simulink model "VSCHVDCunit"  (R2025b)
settings: Solver=VariableStepAuto  StartTime=0.0  StopTime=5  RelTol=1e-3
PreLoadFcn:
  | HVDCParameters;
undefined symbols (not defined in the file): Connection1, Connection2, Connection3, DiscIntNeverNeededParam, ee_sli_rtmsupport, frt, gcbh, grid, HVDC, lvrt, pll, pmsm, PVController, time, Ts, Vdcs0, windController, windTransformer, windTurbine
libraries: nesl_utility x25, fl_lib x24, ee_lib x13, eeGeneralControl x4, eeTransforms x3, simulink x3
(part 1 of 2)
settings Model: SimulationMode=accelerator  Creator=Rajarshi  LastModifiedBy=rajarshd

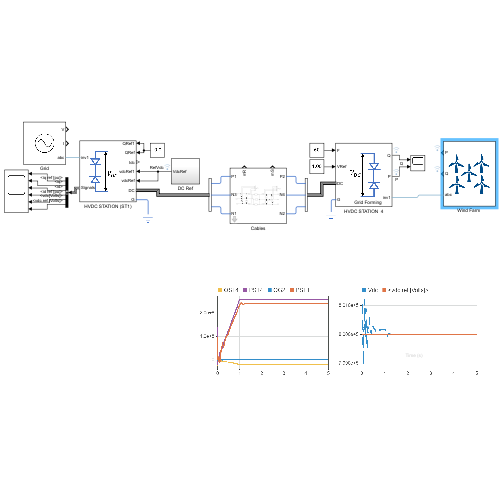
[thumbnail: Simulink's stored preview of the top-level diagram]
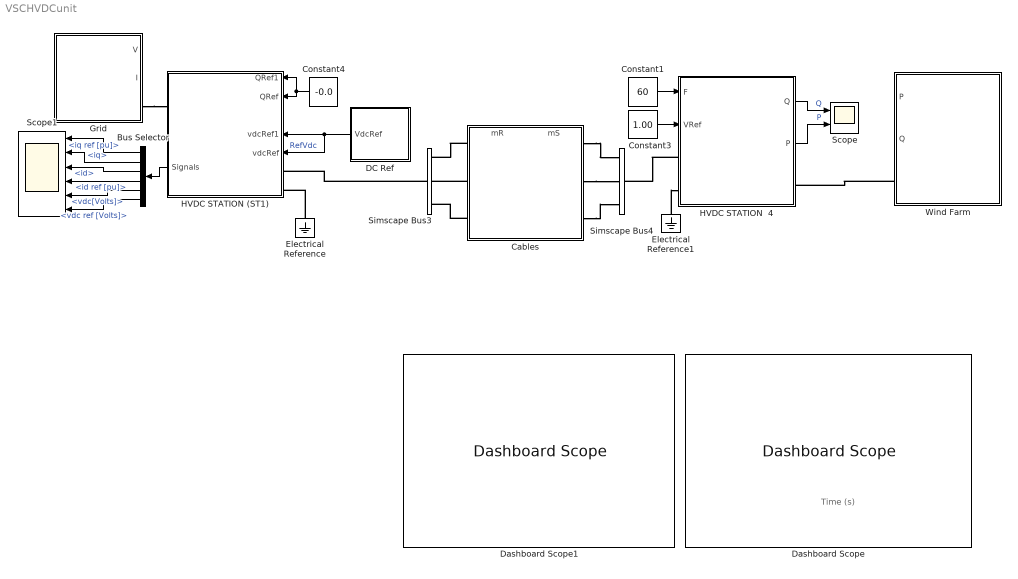
== system VSCHVDCunit ==
  note: Time (s)
  Bus Selector : BusSelector  OutputSignals=iq ref [pu],iq,id,id ref [pu],vdc[Volts],vdc ref [Volts]
  Cables : Subsystem
      settings: PortSchema="{\"entries\":[{\"content\":{\"sides\":[{\"content\":{\"connectorIds\":[\"LConn1\",\"LConn2\",\"LConn3\"]},\"type\":\"ConnectorPlacement.EquallySpacedRectSide\",\"uuid\":\"66d4cfbf-dcba-4749-bf5d-5811a775276e\"},{\"content\":{\"connectorIds\":[\"RConn1\",\"RConn2\",\"RConn3\"],\"side\":\"RIGHT\"},\"type\":\"ConnectorPlacement.EquallySpacedRectSide\",\"uuid\":\"35abdffa-cda0-46f2-9903-3f86a9532248\"},{\"content\":{\"connectorIds\":[\"Out1\",\"Out2\"],\"side\":\"TOP\"},\"type\":\"ConnectorPlacement.EquallySpacedRectSide\",\"uuid\":\"3c5502e5-1b76-444d-b26b-a5789383a319\"},{\"content\":{\"side\":\"BOTTOM\"},\"type\":\"ConnectorPlacement.EquallySpacedRectSide\",\"uuid\":\"683abed6-51b1-463c-bfde-96cc94cb06b2\"}]},\"type\":\"ConnectorPlacement.EquallySpacedConnector\",\"uuid\":\"b78b2c4f-7eb3-43f3-aa61-891430661a3a\"}],\"packageUris\":[\"http://schema.mathworks.com/mf0/Connector/R2020b\"],\"version\":\"1.0\"}"
  Constant1 : Constant  Value=60
  Constant3 : Constant  Value=1.00
  Constant4 : Constant  Value=-0.0
  DC Ref : Subsystem
  Dashboard Scope : DashboardScope  FontColor=[0.0, 0.0, 0.0]
  Dashboard Scope1 : DashboardScope  FontColor=[0.0, 0.0, 0.0]
  Electrical Reference : fl_lib/Electrical/Electrical Elements/Electrical Reference
  Electrical Reference1 : fl_lib/Electrical/Electrical Elements/Electrical Reference
  Grid : Subsystem
  HVDC STATION  4 : Subsystem
      mask Display:
      | text(40,10, 'Grid Forming');
      | image('HVDCstation.png', [0,0,0,0,80,80]);
  HVDC STATION (ST1) : Subsystem
      settings: PortSchema="{\"entries\":[{\"content\":{\"sides\":[{\"content\":{\"connectorIds\":[\"In1\",\"In2\",\"LConn1\",\"In3\",\"In4\",\"LConn2\",\"LConn3\"]},\"type\":\"ConnectorPlacement.EquallySpacedRectSide\",\"uuid\":\"825870e3-6597-48fb-b44e-9cac78187e1c\"},{\"content\":{\"connectorIds\":[\"RConn1\",\"Out1\"],\"side\":\"RIGHT\"},\"type\":\"ConnectorPlacement.EquallySpacedRectSide\",\"uuid\":\"0ccf2e17-8e04-4158-8531-c061fa3c835c\"},{\"content\":{\"side\":\"TOP\"},\"type\":\"ConnectorPlacement.EquallySpacedRectSide\",\"uuid\":\"f5f3d6c6-bb99-4c25-841e-4b6e2b2ba3c2\"}]},\"type\":\"ConnectorPlacement.EquallySpacedConnector\",\"uuid\":\"7882ba9b-b66e-421c-89fd-6c0e858bc84c\"}],\"packageUris\":[\"http://schema.mathworks.com/mf0/Connector/R2020b\"],\"version\":\"1.0\"}"
      mask Display: image('HVDCstation1.png', [0,2,12,2,80,80]);
  Scope : Scope  NumInputPorts=2
      settings: ActiveDisplayYMinimum=-8.229856003977344E+8  ActiveDisplayYMaximum=7.0866847199803662E+8
  Scope1 : Scope  NumInputPorts=6
      settings: ActiveDisplayYMinimum=-0.01126  ActiveDisplayYMaximum=0.00125
  Simscape Bus3 : SimscapeBus  HierarchyStrings=Connection1;Connection2;Connection3
  Simscape Bus4 : SimscapeBus  HierarchyStrings=Connection1;Connection2;Connection3
  "Wind Farm " : Subsystem
      mask Display: image('Windfirm3.png', [0,0,0,0,80,80]);
  wires:
  DC Ref/1(VdcRef) -> HVDC STATION (ST1)/4(vdcRef), HVDC STATION (ST1)/3(vdcRef1)  "RefVdc"
  Constant1/1 -> HVDC STATION  4/1(F)
  Constant4/1 -> HVDC STATION (ST1)/1(QRef1), HVDC STATION (ST1)/2(QRef)
  Constant3/1 -> HVDC STATION  4/2(VRef)
  HVDC STATION (ST1)/1(Signals) -> Bus Selector/1
  Bus Selector/1 -> Scope1/1  "<iq ref [pu]>"
  Bus Selector/2 -> Scope1/2  "<iq>"
  Bus Selector/3 -> Scope1/3  "<id>"
  Bus Selector/4 -> Scope1/4  "<id ref [pu]>"
  Bus Selector/5 -> Scope1/5  "<vdc[Volts]>"
  Bus Selector/6 -> Scope1/6  "<vdc ref [Volts]>"
  HVDC STATION  4/1(Q) -> Scope/1  "Q"
  HVDC STATION  4/2(P) -> Scope/2  "P"
  connections:
  Grid/RConn1 -- HVDC STATION (ST1)/RConn1
  "Wind Farm "/RConn1 -- HVDC STATION  4/RConn1
  Cables/RConn3 -- Simscape Bus4/LConn3
  Cables/LConn1 -- Simscape Bus3/LConn1
  Cables/LConn3 -- Simscape Bus3/LConn3
  Cables/LConn2 -- Simscape Bus3/LConn2
  Cables/RConn2 -- Simscape Bus4/LConn2
  Cables/RConn1 -- Simscape Bus4/LConn1
  HVDC STATION  4/LConn1 -- Simscape Bus4/RConn1
  Simscape Bus3/RConn1 -- HVDC STATION (ST1)/LConn2
  Electrical Reference/LConn1 -- HVDC STATION (ST1)/LConn3
  Electrical Reference1/LConn1 -- HVDC STATION  4/LConn2

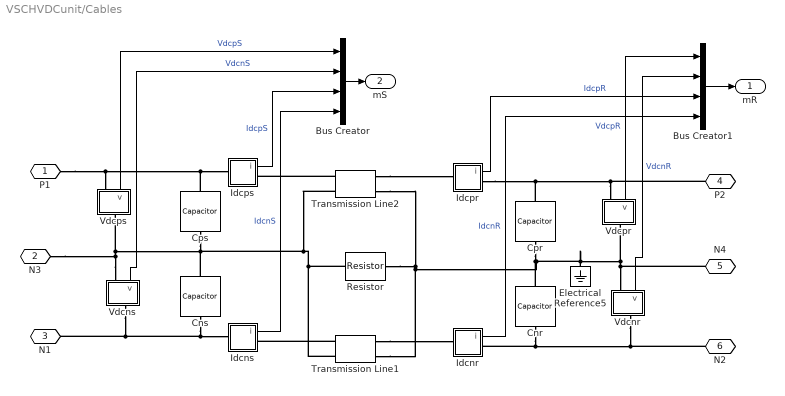
== system VSCHVDCunit/Cables ==
  Bus Creator : BusCreator  Inputs=4
  Bus Creator1 : BusCreator  Inputs=4
  Cnr : fl_lib/Electrical/Electrical Elements/Capacitor  c=0.1e-6 F  r=0 Ohm  g=0 1/Ohm  i_specify=off  i_priority=High  i=0 A  i_nominal_specify=off  i_nominal_value=1  i_nominal_unit=A  v_specify=off  v_priority=High  v=Vdcs0/2 V  v_nominal_specify=off  v_nominal_value=1  v_nominal_unit=V  vc_specify=on  vc_priority=High  vc=HVDC.Vdc V  vc_nominal_specify=off  vc_nominal_value=1  vc_nominal_unit=V
  Cns : fl_lib/Electrical/Electrical Elements/Capacitor  c=0.1e-6 F  r=0 Ohm  g=0 1/Ohm  i_specify=off  i_priority=High  i=0 A  i_nominal_specify=off  i_nominal_value=1  i_nominal_unit=A  v_specify=off  v_priority=High  v=Vdcs0/2 V  v_nominal_specify=off  v_nominal_value=1  v_nominal_unit=V  vc_specify=on  vc_priority=High  vc=HVDC.Vdc V  vc_nominal_specify=off  vc_nominal_value=1  vc_nominal_unit=V
  Cpr : fl_lib/Electrical/Electrical Elements/Capacitor  c=0.1e-6 F  r=0 Ohm  g=0 1/Ohm  i_specify=off  i_priority=High  i=0 A  i_nominal_specify=off  i_nominal_value=1  i_nominal_unit=A  v_specify=off  v_priority=High  v=Vdcs0/2 V  v_nominal_specify=off  v_nominal_value=1  v_nominal_unit=V  vc_specify=on  vc_priority=High  vc=HVDC.Vdc V  vc_nominal_specify=off  vc_nominal_value=1  vc_nominal_unit=V
  Cps : fl_lib/Electrical/Electrical Elements/Capacitor  c=0.1e-6 F  r=0 Ohm  g=0 1/Ohm  i_specify=off  i_priority=High  i=0 A  i_nominal_specify=off  i_nominal_value=1  i_nominal_unit=A  v_specify=off  v_priority=High  v=Vdcs0/2 V  v_nominal_specify=off  v_nominal_value=1  v_nominal_unit=V  vc_specify=on  vc_priority=High  vc=HVDC.Vdc V  vc_nominal_specify=off  vc_nominal_value=1  vc_nominal_unit=V
  Electrical Reference5 : fl_lib/Electrical/Electrical Elements/Electrical Reference
  Idcnr : Subsystem
      settings: PortSchema="{\"entries\":[{\"content\":{\"sides\":[{\"content\":{\"connectorIds\":[\"LConn1\"]},\"type\":\"ConnectorPlacement.EquallySpacedRectSide\",\"uuid\":\"b182dbc5-c8d5-4832-a7cd-ea3787954646\"},{\"content\":{\"connectorIds\":[\"RConn1\",\"Out1\"],\"side\":\"RIGHT\"},\"type\":\"ConnectorPlacement.EquallySpacedRectSide\",\"uuid\":\"bfc6f163-1abf-440b-aa89-1443f971fd07\"},{\"content\":{\"connectorIds\":[],\"side\":\"TOP\"},\"type\":\"ConnectorPlacement.EquallySpacedRectSide\",\"uuid\":\"dd2a104c-9a72-483e-91c4-dbef9b359450\"}]},\"type\":\"ConnectorPlacement.EquallySpacedConnector\",\"uuid\":\"ce98cc3b-f524-409d-a465-fff2e3b7df79\"}],\"packageUris\":[\"http://schema.mathworks.com/mf0/Connector/R2020b\"],\"version\":\"1.0\"}"
  Idcns : Subsystem
      settings: PortSchema="{\"entries\":[{\"content\":{\"sides\":[{\"content\":{\"connectorIds\":[\"LConn1\"]},\"type\":\"ConnectorPlacement.EquallySpacedRectSide\",\"uuid\":\"b182dbc5-c8d5-4832-a7cd-ea3787954646\"},{\"content\":{\"connectorIds\":[\"RConn1\",\"Out1\"],\"side\":\"RIGHT\"},\"type\":\"ConnectorPlacement.EquallySpacedRectSide\",\"uuid\":\"bfc6f163-1abf-440b-aa89-1443f971fd07\"},{\"content\":{\"connectorIds\":[],\"side\":\"TOP\"},\"type\":\"ConnectorPlacement.EquallySpacedRectSide\",\"uuid\":\"dd2a104c-9a72-483e-91c4-dbef9b359450\"}]},\"type\":\"ConnectorPlacement.EquallySpacedConnector\",\"uuid\":\"ce98cc3b-f524-409d-a465-fff2e3b7df79\"}],\"packageUris\":[\"http://schema.mathworks.com/mf0/Connector/R2020b\"],\"version\":\"1.0\"}"
  Idcpr : Subsystem
      settings: PortSchema="{\"entries\":[{\"content\":{\"sides\":[{\"content\":{\"connectorIds\":[\"LConn1\"]},\"type\":\"ConnectorPlacement.EquallySpacedRectSide\",\"uuid\":\"b182dbc5-c8d5-4832-a7cd-ea3787954646\"},{\"content\":{\"connectorIds\":[\"RConn1\",\"Out1\"],\"side\":\"RIGHT\"},\"type\":\"ConnectorPlacement.EquallySpacedRectSide\",\"uuid\":\"bfc6f163-1abf-440b-aa89-1443f971fd07\"},{\"content\":{\"connectorIds\":[],\"side\":\"TOP\"},\"type\":\"ConnectorPlacement.EquallySpacedRectSide\",\"uuid\":\"dd2a104c-9a72-483e-91c4-dbef9b359450\"}]},\"type\":\"ConnectorPlacement.EquallySpacedConnector\",\"uuid\":\"ce98cc3b-f524-409d-a465-fff2e3b7df79\"}],\"packageUris\":[\"http://schema.mathworks.com/mf0/Connector/R2020b\"],\"version\":\"1.0\"}"
  Idcps : Subsystem
      settings: PortSchema="{\"entries\":[{\"content\":{\"sides\":[{\"content\":{\"connectorIds\":[\"LConn1\"]},\"type\":\"ConnectorPlacement.EquallySpacedRectSide\",\"uuid\":\"b182dbc5-c8d5-4832-a7cd-ea3787954646\"},{\"content\":{\"connectorIds\":[\"RConn1\",\"Out1\"],\"side\":\"RIGHT\"},\"type\":\"ConnectorPlacement.EquallySpacedRectSide\",\"uuid\":\"bfc6f163-1abf-440b-aa89-1443f971fd07\"},{\"content\":{\"connectorIds\":[],\"side\":\"TOP\"},\"type\":\"ConnectorPlacement.EquallySpacedRectSide\",\"uuid\":\"dd2a104c-9a72-483e-91c4-dbef9b359450\"}]},\"type\":\"ConnectorPlacement.EquallySpacedConnector\",\"uuid\":\"ce98cc3b-f524-409d-a465-fff2e3b7df79\"}],\"packageUris\":[\"http://schema.mathworks.com/mf0/Connector/R2020b\"],\"version\":\"1.0\"}"
  Resistor : fl_lib/Electrical/Electrical Elements/Resistor  R=125*1e-5 Ohm  i_specify=off  i_priority=None  i=0 A  i_nominal_specify=off  i_nominal_value=1  i_nominal_unit=A  v_specify=off  v_priority=None  v=0 V  v_nominal_specify=off  v_nominal_value=1  v_nominal_unit=V
  Transmission Line1 : ee_lib/Passive/Lines/Transmission Line  model_type=4  TD=5 ns  LC_param=2  Z0_delay_based=50 Ohm  Z0=50 Ohm  freq=60 Hz  Ll=0.47/1000 mH/m  L=2.1120/1000 mH/m  C=0.1906/1000 uF/m  R=0.0095/1000 Ohm/m  G=0.048 /1000 uS/m  LEN=125 km  N=1
      settings: InternalSimscapePortConfiguration="{\"Bottom\":[],\"Left\":[{\"id\":\"p1\",\"label\":\"\",\"type\":\"foundation.electrical.electrical\"},{\"id\":\"n1\",\"label\":\"\",\"type\":\"foundation.electrical.electrical\"}],\"Right\":[{\"id\":\"p2\",\"label\":\"\",\"type\":\"foundation.electrical.electrical\"},{\"id\":\"n2\",\"label\":\"\",\"type\":\"foundation.electrical.electrical\"}],\"Top\":[]}"
  Transmission Line2 : ee_lib/Passive/Lines/Transmission Line  model_type=4  TD=5 ns  LC_param=2  Z0_delay_based=50 Ohm  Z0=50 Ohm  freq=60 Hz  Ll=0.47/1000 mH/m  L=2.1120/1000 mH/m  C=0.1906/1000 uF/m  R=0.0095/1000 Ohm/m  G=0.048/1000 uS/m  LEN=125 km  N=1
      settings: InternalSimscapePortConfiguration="{\"Bottom\":[],\"Left\":[{\"id\":\"p1\",\"label\":\"\",\"type\":\"foundation.electrical.electrical\"},{\"id\":\"n1\",\"label\":\"\",\"type\":\"foundation.electrical.electrical\"}],\"Right\":[{\"id\":\"p2\",\"label\":\"\",\"type\":\"foundation.electrical.electrical\"},{\"id\":\"n2\",\"label\":\"\",\"type\":\"foundation.electrical.electrical\"}],\"Top\":[]}"
  Vdcnr : Subsystem
      settings: PortSchema="{\"entries\":[{\"content\":{\"sides\":[{\"content\":{\"connectorIds\":[\"LConn1\",\"Out1\"]},\"type\":\"ConnectorPlacement.EquallySpacedRectSide\",\"uuid\":\"bc3757cc-4537-444e-89af-7b7d8c8c1fa7\"},{\"content\":{\"connectorIds\":[\"RConn1\"],\"side\":\"RIGHT\"},\"type\":\"ConnectorPlacement.EquallySpacedRectSide\",\"uuid\":\"908bf4c4-26f6-4d8a-bcf8-68236027f5f8\"},{\"content\":{\"side\":\"TOP\"},\"type\":\"ConnectorPlacement.EquallySpacedRectSide\",\"uuid\":\"33f228db-ba47-4718-96dc-a72de309ae8c\"},{\"content\":{\"side\":\"BOTTOM\"},\"type\":\"ConnectorPlacement.EquallySpacedRectSide\",\"uuid\":\"d9b66c7e-0954-4c47-8bcc-77bf13ff573c\"}]},\"type\":\"ConnectorPlacement.EquallySpacedConnector\",\"uuid\":\"345f3578-0572-4e64-b2f3-84728129a12d\"}],\"packageUris\":[\"http://schema.mathworks.com/mf0/Connector/R2020b\"],\"version\":\"1.0\"}"
  Vdcns : Subsystem
      settings: PortSchema="{\"entries\":[{\"content\":{\"sides\":[{\"content\":{\"connectorIds\":[\"LConn1\",\"Out1\"]},\"type\":\"ConnectorPlacement.EquallySpacedRectSide\",\"uuid\":\"bc3757cc-4537-444e-89af-7b7d8c8c1fa7\"},{\"content\":{\"connectorIds\":[\"RConn1\"],\"side\":\"RIGHT\"},\"type\":\"ConnectorPlacement.EquallySpacedRectSide\",\"uuid\":\"908bf4c4-26f6-4d8a-bcf8-68236027f5f8\"},{\"content\":{\"side\":\"TOP\"},\"type\":\"ConnectorPlacement.EquallySpacedRectSide\",\"uuid\":\"33f228db-ba47-4718-96dc-a72de309ae8c\"},{\"content\":{\"side\":\"BOTTOM\"},\"type\":\"ConnectorPlacement.EquallySpacedRectSide\",\"uuid\":\"d9b66c7e-0954-4c47-8bcc-77bf13ff573c\"}]},\"type\":\"ConnectorPlacement.EquallySpacedConnector\",\"uuid\":\"345f3578-0572-4e64-b2f3-84728129a12d\"}],\"packageUris\":[\"http://schema.mathworks.com/mf0/Connector/R2020b\"],\"version\":\"1.0\"}"
  Vdcpr : Subsystem
      settings: PortSchema="{\"entries\":[{\"content\":{\"sides\":[{\"content\":{\"connectorIds\":[\"LConn1\",\"Out1\"]},\"type\":\"ConnectorPlacement.EquallySpacedRectSide\",\"uuid\":\"bc3757cc-4537-444e-89af-7b7d8c8c1fa7\"},{\"content\":{\"connectorIds\":[\"RConn1\"],\"side\":\"RIGHT\"},\"type\":\"ConnectorPlacement.EquallySpacedRectSide\",\"uuid\":\"908bf4c4-26f6-4d8a-bcf8-68236027f5f8\"},{\"content\":{\"side\":\"TOP\"},\"type\":\"ConnectorPlacement.EquallySpacedRectSide\",\"uuid\":\"33f228db-ba47-4718-96dc-a72de309ae8c\"},{\"content\":{\"side\":\"BOTTOM\"},\"type\":\"ConnectorPlacement.EquallySpacedRectSide\",\"uuid\":\"d9b66c7e-0954-4c47-8bcc-77bf13ff573c\"}]},\"type\":\"ConnectorPlacement.EquallySpacedConnector\",\"uuid\":\"345f3578-0572-4e64-b2f3-84728129a12d\"}],\"packageUris\":[\"http://schema.mathworks.com/mf0/Connector/R2020b\"],\"version\":\"1.0\"}"
  Vdcps : Subsystem
      settings: PortSchema="{\"entries\":[{\"content\":{\"sides\":[{\"content\":{\"connectorIds\":[\"LConn1\",\"Out1\"]},\"type\":\"ConnectorPlacement.EquallySpacedRectSide\",\"uuid\":\"bc3757cc-4537-444e-89af-7b7d8c8c1fa7\"},{\"content\":{\"connectorIds\":[\"RConn1\"],\"side\":\"RIGHT\"},\"type\":\"ConnectorPlacement.EquallySpacedRectSide\",\"uuid\":\"908bf4c4-26f6-4d8a-bcf8-68236027f5f8\"},{\"content\":{\"side\":\"TOP\"},\"type\":\"ConnectorPlacement.EquallySpacedRectSide\",\"uuid\":\"33f228db-ba47-4718-96dc-a72de309ae8c\"},{\"content\":{\"side\":\"BOTTOM\"},\"type\":\"ConnectorPlacement.EquallySpacedRectSide\",\"uuid\":\"d9b66c7e-0954-4c47-8bcc-77bf13ff573c\"}]},\"type\":\"ConnectorPlacement.EquallySpacedConnector\",\"uuid\":\"345f3578-0572-4e64-b2f3-84728129a12d\"}],\"packageUris\":[\"http://schema.mathworks.com/mf0/Connector/R2020b\"],\"version\":\"1.0\"}"
  P1 : PMIOPort  Side=Left
  N3 : PMIOPort  Port=2  Side=Left
  N1 : PMIOPort  Port=3  Side=Left
  P2 : PMIOPort  Port=4  Side=Right
  N4 : PMIOPort  Port=5  Side=Right
  N2 : PMIOPort  Port=6  Side=Right
  mR : Outport
  mS : Outport  Port=2
  wires:
  Vdcps/1(v) -> Bus Creator/1  "VdcpS"
  Vdcns/1(v) -> Bus Creator/2  "VdcnS"
  Idcps/1(i) -> Bus Creator/3  "IdcpS"
  Idcns/1(i) -> Bus Creator/4  "IdcnS"
  Bus Creator/1 -> mS/1
  Bus Creator1/1 -> mR/1
  Idcnr/1(i) -> Bus Creator1/4  "IdcnR"
  Idcpr/1(i) -> Bus Creator1/3  "IdcpR"
  Vdcpr/1(v) -> Bus Creator1/1  "VdcpR"
  Vdcnr/1(v) -> Bus Creator1/2  "VdcnR"
  connections:
  P1/RConn1 -- Idcps/LConn1 -- Cps/LConn1 -- Vdcps/LConn1
  Cns/RConn1 -- Idcns/LConn1 -- Vdcns/RConn1 -- N1/RConn1
  Vdcns/LConn1 -- Vdcps/RConn1 -- Resistor/LConn1 -- Transmission Line1/LConn2 -- Transmission Line2/LConn2 -- Cps/RConn1 -- Cns/LConn1 -- N3/RConn1
  Cpr/RConn1 -- Resistor/RConn1 -- Transmission Line2/RConn2 -- Transmission Line1/RConn2 -- N4/RConn1 -- Vdcnr/LConn1 -- Vdcpr/RConn1 -- Electrical Reference5/LConn1 -- Cnr/LConn1
  Cnr/RConn1 -- Idcnr/RConn1 -- N2/RConn1 -- Vdcnr/RConn1
  Vdcpr/LConn1 -- P2/RConn1 -- Cpr/LConn1 -- Idcpr/RConn1
  Transmission Line2/LConn1 -- Idcps/RConn1
  Transmission Line2/RConn1 -- Idcpr/LConn1
  Transmission Line1/LConn1 -- Idcns/RConn1
  Transmission Line1/RConn1 -- Idcnr/LConn1

== system VSCHVDCunit/DC Ref ==
  Constant : Constant  Value=HVDC.Vdc
  Gain1 : Gain  Gain=2
  Terminator1 : Terminator
  VdcRef : Outport
  wires:
  Constant/1 -> VdcRef/1, Gain1/1
  Gain1/1 -> Terminator1/1  "VdcRef"

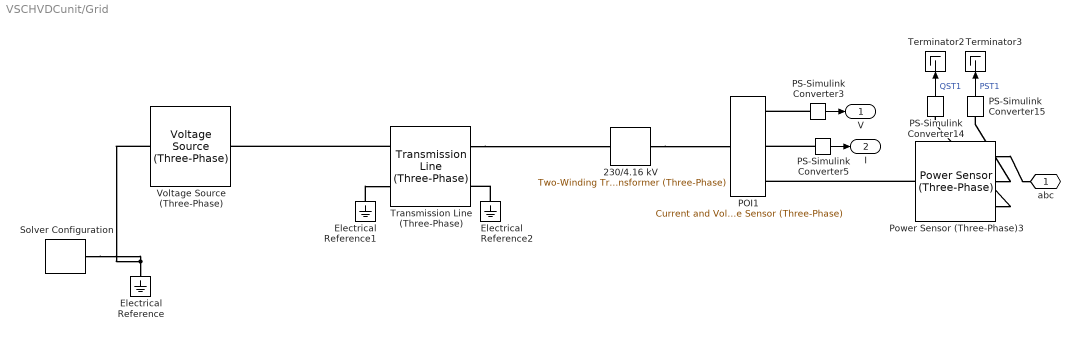
== system VSCHVDCunit/Grid ==
  230/4.16 kV : ee_lib/Passive/Transformers/Two-Winding Transformer (Three-Phase)  SRated=windTransformer.va A*V  FRated=grid.frequency Hz  Winding1Connection=ee.enum.windingconnection.Yg  VRated1=windTransformer.hv V  Winding2Connection=ee.enum.windingconnection.Yg  VRated2=base.kV V  CoreType=ee.enum.coretype.threelimb  pu_Rw1=windTransformer.windingResistance/20  pu_Rw2=windTransformer.windingResistance/20  leakage_reactance_option=ee.enum.transformer_leakage.include  pu_Xl1=windTransformer.windingLekageReactance/20  pu_Xl2=windTransformer.windingLekageReactance/20  magnetizing_resistance_option=ee.enum.transformer_magnetizingResistance.exclude  pu_Rm=500  magnetizing_reactance_option=ee.enum.transformer_magnetizingReactance.exclude  saturation_option=ee.enum.transformer_saturation.exclude  pu_Xm=500  current_data=[0, .002, 1, 2]  magnetic_flux_data=[0, 1.2, 1.5, 1.51]  pu_X0=windTransformer.zeroSequenceReactance  i1_specify=off  i1_priority=None  i1=[0, 0, 0] A  i1_nominal_specify=off  i1_nominal_value=1  i1_nominal_unit=A  i2_specify=off  i2_priority=None  i2=[0, 0, 0] A  i2_nominal_specify=off  i2_nominal_value=1  i2_nominal_unit=A  phi_specify=off  phi_priority=None  phi=[0, 0, 0]  phi_nominal_specify=off  phi_nominal_value=1  phi_nominal_unit=1  power_dissipated_specify=off  power_dissipated_priority=None  power_dissipated=0 W  power_dissipated_nominal_specify=off  power_dissipated_nominal_value=1  power_dissipated_nominal_unit=W
      settings: InternalSimscapePortConfiguration="{\"Bottom\":[],\"Left\":[{\"id\":\"N1\",\"label\":\"~1\",\"type\":\"foundation.electrical.three_phase\"}],\"Right\":[{\"id\":\"N2\",\"label\":\"~2\",\"type\":\"foundation.electrical.three_phase\"}],\"Top\":[]}"
  Electrical Reference : fl_lib/Electrical/Electrical Elements/Electrical Reference
  Electrical Reference1 : fl_lib/Electrical/Electrical Elements/Electrical Reference
  Electrical Reference2 : fl_lib/Electrical/Electrical Elements/Electrical Reference
  POI1 : ee_lib/Sensors & Transducers/Current and Voltage Sensor (Three-Phase)  vMeasurementType=ee.enum.vmeasurement.lg  outputUnit=ee.enum.unit.pu  SRated=Base.MVA_base_new A*V  VRated=66e3 V  I_specify=off  I_priority=None  I=[0, 0, 0] A  I_nominal_specify=off  I_nominal_value=1  I_nominal_unit=A  V_specify=off  V_priority=None  V=[0, 0, 0] V  V_nominal_specify=off  V_nominal_value=1  V_nominal_unit=V
      settings: InternalSimscapePortConfiguration="{\"Bottom\":[],\"Left\":[{\"id\":\"N1\",\"label\":\"~1\",\"type\":\"foundation.electrical.three_phase\"}],\"Right\":[{\"id\":\"V_output\",\"label\":\"V\",\"type\":\"output\"},{\"id\":\"I_output\",\"label\":\"I\",\"type\":\"output\"},{\"id\":\"N2\",\"label\":\"~2\",\"type\":\"foundation.electrical.three_phase\"}],\"Top\":[]}"
  PS-Simulink Converter{3,5,14..15} (4 alike) : nesl_utility/PS-Simulink Converter  PhysicalDomain=network_engine_domain  SubClassName=ps_output  LeftPortType=input  RightPortType=output  PseudoPeriodic=off  Frequencies=[]  VectorFormat=inherit  Unit=inherit  AffineConversion=off
  Power Sensor (Three-Phase)3 : ee_lib/Sensors & Transducers/Power Sensor (Three-Phase)  load_type=ee.enum.passive.type_balanced.balanced  f0=60 Hz
      settings: InternalSimscapePortConfiguration="{\"Bottom\":[],\"Left\":[{\"id\":\"N1\",\"label\":\"~1\",\"type\":\"foundation.electrical.three_phase\"}],\"Right\":[{\"id\":\"N2\",\"label\":\"~2\",\"type\":\"foundation.electrical.three_phase\"}],\"Top\":[{\"id\":\"Pm\",\"label\":\"P\",\"type\":\"output\"},{\"id\":\"Qm\",\"label\":\"Q\",\"type\":\"output\"}]}"
  Solver Configuration : nesl_utility/Solver Configuration  PhysicalDomain=network_engine_domain  SubClassName=solver  LeftPortType=input  RightPortType=generic  Tones=[]  Harmonics=[]  SimulateNoise=off  Profile=off  UseLocalSampling=off  EnableSwitchedLinearOptims=on  FrequencyDomain=off  UseCCode=off  RelTol=0.001  AbsTol=0.001  MinStep=1e-09  ToWorkspace=off  RevertToSquareIcSolve=off  NumHomotopyIterations=100  PhasorMode=off  PhasorModeNumHarmonics=1  ConsistencySolver=NEWTON_XTOL_AFTER_FTOL  IndexReductionMethod=None  DoDC=off  ResidualTolerance=1e-09  ConsistencyTolSource=LOCAL  ConsistencyAbsTol=1e5  ConsistencyRelTol=1e5  ConsistencyTolFactor=1e5  UseLocalSolver=on  LocalSolverChoice=NE_BACKWARD_EULER_ADVANCER  ResolveIndetEquations=on  FunctionEvalNumThread=1  LocalSolverSampleTime=5e-5  DoFixedCost=on  MaxNonlinIter=1  MaxModeIter=2  ComputeImpulses=off  ImpulseIterations=2  LinearAlgebra=Sparse  LinearAlgebraNumThread=0  EquationFormulation=NE_TIME_EF  DelaysMemoryBudget=1024  AutomaticFiltering=off  FilteringTimeConstant=0.001  PartitionStorageMethod=AS_NEEDED  PartitionMemoryBudget=1024  PartitionMethod=ROBUST  MultibodyUseLocalSolver=off  MultibodyLocalSolverChoice=ODE1  MultibodyLocalSolverSampleTime=0.001
  Terminator2 : Terminator
  Terminator3 : Terminator
  Transmission Line (Three-Phase) : ee_lib/Passive/Lines/Transmission Line (Three-Phase)  length=10 km  freq=60 Hz  R=0.02 Ohm/km  L=0.5 mH/km  M=0.1 mH/km  Cl=0.3 uF/km  Cg=0.1 uF/km  Rm=0 Ohm/km  ModelTwoSections=ee.enum.enable.no  N=1  InterfacePosition=0.5 km  N1sec=1  N2sec=1  Access_ground=ee.enum.enable.no  R_parasitic=1e-6 Ohm  G_parasitic=1e-6 1/Ohm
      settings: InternalSimscapePortConfiguration="{\"Bottom\":[],\"Left\":[{\"id\":\"N1\",\"label\":\"~1\",\"type\":\"foundation.electrical.three_phase\"},{\"id\":\"g1\",\"label\":\"g1\",\"type\":\"foundation.electrical.electrical\"}],\"Right\":[{\"id\":\"N2\",\"label\":\"~2\",\"type\":\"foundation.electrical.three_phase\"},{\"id\":\"g2\",\"label\":\"g2\",\"type\":\"foundation.electrical.electrical\"}],\"Top\":[]}"
  Voltage Source (Three-Phase) : ee_lib/Sources/Voltage Source (Three-Phase)  vline_rms=230e3 V  shift=0 deg  freq=60 Hz  impedance_option=0  SShortCircuit=1e6 A*V  XR=15  R=0.01 Ohm  L=3.97e-4 H  harmonic_option=0  harmonic_orders=[5, 7, 11, 13]  harmonic_ratios=[.1, .1, .1, .1]  G_parasitic=0 1/Ohm  I_specify=off  I_priority=None  I=[0, 0, 0] A  I_nominal_specify=off  I_nominal_value=1  I_nominal_unit=A
  abc : PMIOPort  Side=Right
  V : Outport
  I : Outport  Port=2
  wires:
  PS-Simulink Converter3/1 -> V/1
  PS-Simulink Converter5/1 -> I/1
  PS-Simulink Converter14/1 -> Terminator2/1  "QST1"
  PS-Simulink Converter15/1 -> Terminator3/1  "PST1"
  connections:
  230/4.16 kV/RConn1 -- POI1/LConn1
  PS-Simulink Converter3/LConn1 -- POI1/RConn1
  PS-Simulink Converter5/LConn1 -- POI1/RConn2
  Power Sensor (Three-Phase)3/LConn2 -- PS-Simulink Converter15/LConn1
  Power Sensor (Three-Phase)3/LConn3 -- PS-Simulink Converter14/LConn1
  Power Sensor (Three-Phase)3/LConn1 -- abc/RConn1
  Power Sensor (Three-Phase)3/RConn1 -- POI1/RConn3
  Electrical Reference/LConn1 -- Voltage Source (Three-Phase)/LConn1 -- Solver Configuration/RConn1
  Electrical Reference1/LConn1 -- Transmission Line (Three-Phase)/LConn2
  Electrical Reference2/LConn1 -- Transmission Line (Three-Phase)/RConn2
  Transmission Line (Three-Phase)/LConn1 -- Voltage Source (Three-Phase)/RConn1
  Transmission Line (Three-Phase)/RConn1 -- 230/4.16 kV/LConn1

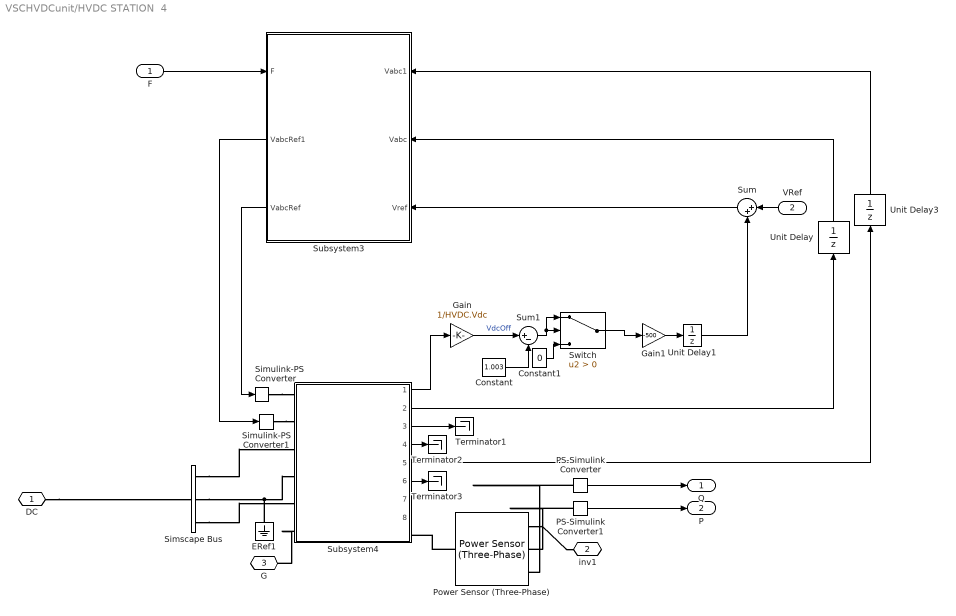
== system VSCHVDCunit/HVDC STATION  4 ==
  F : Inport
  VRef : Inport  Port=2
  Constant : Constant  Value=1.003
  Constant1 : Constant  Value=0
  ERef1 : fl_lib/Electrical/Electrical Elements/Electrical Reference
  Gain : Gain  Gain=1/HVDC.Vdc
  Gain1 : Gain  Gain=-500
  PS-Simulink Converter : nesl_utility/PS-Simulink Converter  PhysicalDomain=network_engine_domain  SubClassName=ps_output  LeftPortType=input  RightPortType=output  PseudoPeriodic=off  Frequencies=[]  VectorFormat=inherit  Unit=inherit  AffineConversion=off
  PS-Simulink Converter1 : nesl_utility/PS-Simulink Converter  PhysicalDomain=network_engine_domain  SubClassName=ps_output  LeftPortType=input  RightPortType=output  PseudoPeriodic=off  Frequencies=[]  VectorFormat=inherit  Unit=inherit  AffineConversion=off
  Power Sensor (Three-Phase) : ee_lib/Sensors & Transducers/Power Sensor (Three-Phase)  load_type=ee.enum.passive.type_balanced.balanced  f0=60 Hz
      settings: InternalSimscapePortConfiguration="{\"Bottom\":[],\"Left\":[{\"id\":\"N1\",\"label\":\"~1\",\"type\":\"foundation.electrical.three_phase\"}],\"Right\":[{\"id\":\"N2\",\"label\":\"~2\",\"type\":\"foundation.electrical.three_phase\"}],\"Top\":[{\"id\":\"Pm\",\"label\":\"P\",\"type\":\"output\"},{\"id\":\"Qm\",\"label\":\"Q\",\"type\":\"output\"}]}"
  Simscape Bus : SimscapeBus  HierarchyStrings=Connection1;Connection2;Connection3
  Simulink-PS Converter : nesl_utility/Simulink-PS Converter  PhysicalDomain=network_engine_domain  SubClassName=ps_input  LeftPortType=input  RightPortType=output  PseudoPeriodic=off  Frequencies=[]  NoiseDistribution=none  NoiseParameters=[]  Unit=1  AffineConversion=off  FilteringAndDerivatives=provide  SimscapeFilterOrder=1  InputFilterTimeConstant=0.001  UdotUserProvided=0
  Simulink-PS Converter1 : nesl_utility/Simulink-PS Converter  PhysicalDomain=network_engine_domain  SubClassName=ps_input  LeftPortType=input  RightPortType=output  PseudoPeriodic=off  Frequencies=[]  NoiseDistribution=none  NoiseParameters=[]  Unit=1  AffineConversion=off  FilteringAndDerivatives=provide  SimscapeFilterOrder=1  InputFilterTimeConstant=0.001  UdotUserProvided=0
  Subsystem3 : Subsystem
      settings: PortSchema="{\"entries\":[{\"content\":{\"sides\":[{\"content\":{\"connectorIds\":[\"In1\",\"In2\",\"In3\"]},\"type\":\"ConnectorPlacement.EquallySpacedRectSide\",\"uuid\":\"fdf47ade-06a3-4164-a0ae-b5ab8f0b8a55\"},{\"content\":{\"connectorIds\":[\"In4\",\"Out1\",\"Out2\"],\"side\":\"RIGHT\"},\"type\":\"ConnectorPlacement.EquallySpacedRectSide\",\"uuid\":\"e0a966ff-b656-4cbf-a7ff-a400da725053\"},{\"content\":{\"side\":\"TOP\"},\"type\":\"ConnectorPlacement.EquallySpacedRectSide\",\"uuid\":\"151062ed-8c36-492f-8148-99554d7644ec\"},{\"content\":{\"side\":\"BOTTOM\"},\"type\":\"ConnectorPlacement.EquallySpacedRectSide\",\"uuid\":\"8f8a2450-c04a-404e-aef9-a0f993b87536\"}]},\"type\":\"ConnectorPlacement.EquallySpacedConnector\",\"uuid\":\"01811104-26cd-432b-92b8-9bb1e91d8204\"}],\"packageUris\":[\"http://schema.mathworks.com/mf0/Connector/R2020b\"],\"version\":\"1.0\"}"
  Subsystem4 : Subsystem  ReferencedSubsystem=HVDCSTATION  c=HVDC.C*0.1  vc=HVDC.Vdc  L=HVDC.L/5  VRated=base.kV1  SRated=Base.MVA_base_new  t=grid.sensorTime  Ts=Ts
  Sum : Sum  Inputs=|++
  Sum1 : Sum  Inputs=|+-
  Switch : Switch  Criteria=u2 > Threshold  SaturateOnIntegerOverflow=off  InputSameDT=off
  Terminator1 : Terminator
  Terminator2 : Terminator
  Terminator3 : Terminator
  Unit Delay : UnitDelay  SampleTime=-1  HasFrameUpgradeWarning=on
  Unit Delay1 : UnitDelay  SampleTime=-1  HasFrameUpgradeWarning=on
  Unit Delay3 : UnitDelay  SampleTime=-1  HasFrameUpgradeWarning=on
  DC : PMIOPort  Side=Left
  inv1 : PMIOPort  Port=2  Side=Right
  G : PMIOPort  Port=3  Side=Left
  Q : Outport
  P : Outport  Port=2
  wires:
  Subsystem4/2 -> Unit Delay/1
  Subsystem4/6 -> Terminator3/1
  Subsystem4/5 -> Unit Delay3/1
  Subsystem4/4 -> Terminator2/1
  F/1 -> Subsystem3/4(F)
  Subsystem4/3 -> Terminator1/1
  Sum/1 -> Subsystem3/3(Vref)
  VRef/1 -> Sum/1
  PS-Simulink Converter1/1 -> P/1
  PS-Simulink Converter/1 -> Q/1
  Unit Delay/1 -> Subsystem3/2(Vabc)
  Unit Delay3/1 -> Subsystem3/1(Vabc1)
  Gain/1 -> Sum1/1  "VdcOff"
  Constant/1 -> Sum1/2
  Constant1/1 -> Switch/3
  Switch/1 -> Gain1/1
  Sum1/1 -> Switch/1, Switch/2
  Gain1/1 -> Unit Delay1/1
  Unit Delay1/1 -> Sum/2
  Subsystem4/1 -> Gain/1
  Subsystem3/2(VabcRef) -> Simulink-PS Converter/1
  Subsystem3/1(VabcRef1) -> Simulink-PS Converter1/1
  connections:
  DC/RConn1 -- Simscape Bus/RConn1
  PS-Simulink Converter/LConn1 -- Power Sensor (Three-Phase)/LConn3
  Power Sensor (Three-Phase)/LConn1 -- inv1/RConn1
  Power Sensor (Three-Phase)/RConn1 -- Subsystem4/RConn1
  PS-Simulink Converter1/LConn1 -- Power Sensor (Three-Phase)/LConn2
  ERef1/LConn1 -- Subsystem4/LConn4 -- Simscape Bus/LConn2
  Simscape Bus/LConn1 -- Subsystem4/LConn3
  Simscape Bus/LConn3 -- Subsystem4/LConn5
  Subsystem4/LConn6 -- G/RConn1
  Simulink-PS Converter/RConn1 -- Subsystem4/LConn1
  Simulink-PS Converter1/RConn1 -- Subsystem4/LConn2

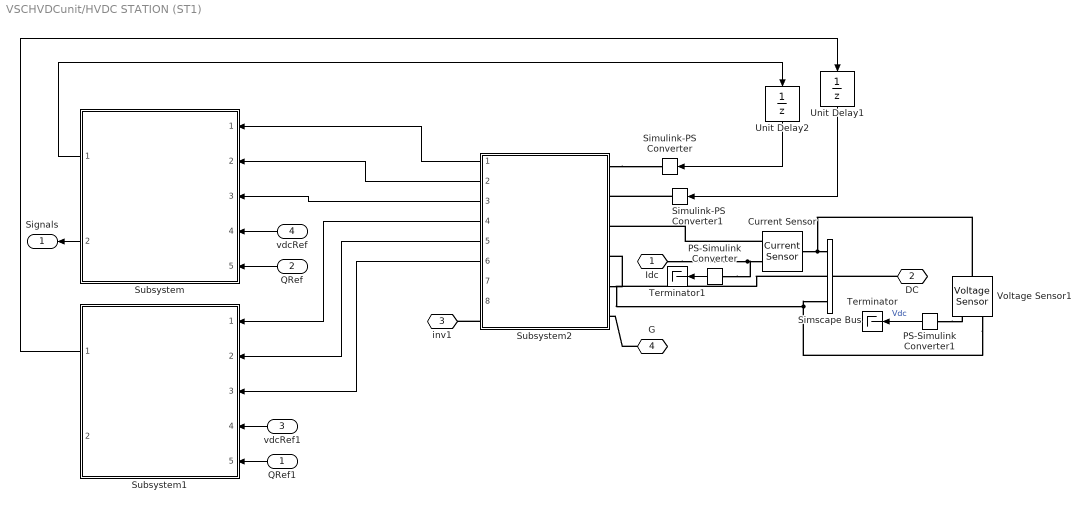
== system VSCHVDCunit/HVDC STATION (ST1) ==
  QRef1 : Inport
  QRef : Inport  Port=2
  vdcRef1 : Inport  Port=3
  vdcRef : Inport  Port=4
  Current Sensor : fl_lib/Electrical/Electrical Sensors/Current Sensor
  PS-Simulink Converter : nesl_utility/PS-Simulink Converter  PhysicalDomain=network_engine_domain  SubClassName=ps_output  LeftPortType=input  RightPortType=output  PseudoPeriodic=off  Frequencies=[]  VectorFormat=inherit  Unit=inherit  AffineConversion=off
  PS-Simulink Converter1 : nesl_utility/PS-Simulink Converter  PhysicalDomain=network_engine_domain  SubClassName=ps_output  LeftPortType=input  RightPortType=output  PseudoPeriodic=off  Frequencies=[]  VectorFormat=inherit  Unit=inherit  AffineConversion=off
  Simscape Bus : SimscapeBus  HierarchyStrings=Connection1;Connection2;Connection3
  Simulink-PS Converter : nesl_utility/Simulink-PS Converter  PhysicalDomain=network_engine_domain  SubClassName=ps_input  LeftPortType=input  RightPortType=output  PseudoPeriodic=off  Frequencies=[]  NoiseDistribution=none  NoiseParameters=[]  Unit=1  AffineConversion=off  FilteringAndDerivatives=provide  SimscapeFilterOrder=1  InputFilterTimeConstant=0.001  UdotUserProvided=0
  Simulink-PS Converter1 : nesl_utility/Simulink-PS Converter  PhysicalDomain=network_engine_domain  SubClassName=ps_input  LeftPortType=input  RightPortType=output  PseudoPeriodic=off  Frequencies=[]  NoiseDistribution=none  NoiseParameters=[]  Unit=1  AffineConversion=off  FilteringAndDerivatives=provide  SimscapeFilterOrder=1  InputFilterTimeConstant=0.001  UdotUserProvided=0
  Subsystem : Subsystem  ReferencedSubsystem=DCVoltageControl  Kppll=PLL.Kp_pll  Kipll=PLL.Ki_pll  frequency=Grid.frequency  initialPhase=0  sampleTime=-1  Kpicd=PVController.Kp_ic*1.02  Kiicd=PVController.Ki_ic*10  Kdicd=.5  Kpicq=PVController.Kp_ic  Kiicq=PVController.Ki_ic*10  Kdicq=.5  Kpv=2  Kiv=1000  Kdv=0  L=HVDC.L*5  iMax=HVDC.Imaxpu  zBase=Base.z_base  mVAbase=Base.MVA_base_new  VdcBase=HVDC.Vdcbase
  Subsystem1 : Subsystem  ReferencedSubsystem=DCVoltageControl  Kppll=PLL.Kp_pll  Kipll=PLL.Ki_pll  frequency=Grid.frequency  initialPhase=0  sampleTime=-1  Kpicd=PVController.Kp_ic*1.02  Kiicd=PVController.Ki_ic*10  Kdicd=0.5  Kpicq=PVController.Kp_ic  Kiicq=PVController.Ki_ic*10  Kdicq=0.5  Kpv=2  Kiv=2000  Kdv=0  L=HVDC.L*100  iMax=HVDC.Imaxpu  zBase=Base.z_base  mVAbase=Base.MVA_base_new  VdcBase=HVDC.Vdcbase
  Subsystem2 : Subsystem  ReferencedSubsystem=HVDCSTATION  c=HVDC.C*0.175  vc=HVDC.Vdc  L=HVDC.L*100  VRated=Base.KV_base_new  SRated=Base.MVA_base_new  t=Grid.sensor_time  Ts=Ts
  Terminator : Terminator
  Terminator1 : Terminator
  Unit Delay1 : UnitDelay  SampleTime=Ts  HasFrameUpgradeWarning=on
  Unit Delay2 : UnitDelay  SampleTime=Ts  HasFrameUpgradeWarning=on
  Voltage Sensor1 : fl_lib/Electrical/Electrical Sensors/Voltage Sensor
  Idc : PMIOPort  Side=Left
  DC : PMIOPort  Port=2  Side=Left
  inv1 : PMIOPort  Port=3  Side=Right
  G : PMIOPort  Port=4  Side=Left
  Signals : Outport
  wires:
  PS-Simulink Converter1/1 -> Terminator/1  "Vdc"
  Subsystem/1 -> Unit Delay2/1
  Subsystem1/1 -> Unit Delay1/1
  vdcRef/1 -> Subsystem/4
  QRef/1 -> Subsystem/5
  vdcRef1/1 -> Subsystem1/4
  QRef1/1 -> Subsystem1/5
  Subsystem2/1 -> Subsystem/1
  Subsystem2/2 -> Subsystem/2
  Subsystem2/3 -> Subsystem/3
  Subsystem2/4 -> Subsystem1/1
  Subsystem2/5 -> Subsystem1/2
  Subsystem2/6 -> Subsystem1/3
  PS-Simulink Converter/1 -> Terminator1/1
  Subsystem/2 -> Signals/1
  Unit Delay2/1 -> Simulink-PS Converter/1
  Unit Delay1/1 -> Simulink-PS Converter1/1
  connections:
  Subsystem2/RConn1 -- inv1/RConn1
  PS-Simulink Converter1/LConn1 -- Voltage Sensor1/RConn1
  DC/RConn1 -- Simscape Bus/RConn1
  Current Sensor/LConn1 -- Voltage Sensor1/LConn1 -- Simscape Bus/LConn1
  Idc/RConn1 -- PS-Simulink Converter/LConn1 -- Current Sensor/RConn1
  Voltage Sensor1/RConn2 -- Subsystem2/LConn5 -- Simscape Bus/LConn3
  Subsystem2/LConn1 -- Simulink-PS Converter/RConn1
  Simulink-PS Converter1/RConn1 -- Subsystem2/LConn2
  Current Sensor/RConn2 -- Subsystem2/LConn3
  Simscape Bus/LConn2 -- Subsystem2/LConn4
  G/RConn1 -- Subsystem2/LConn6

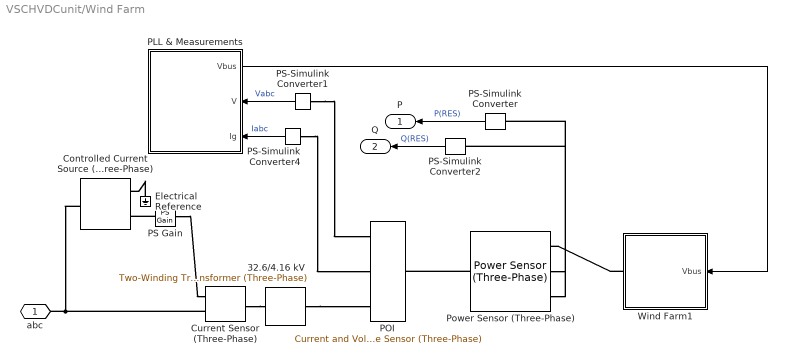
== system VSCHVDCunit/Wind Farm  ==
  32.6/4.16 kV : ee_lib/Passive/Transformers/Two-Winding Transformer (Three-Phase)  SRated=windTransformer.va A*V  FRated=grid.frequency Hz  Winding1Connection=ee.enum.windingconnection.Yg  VRated1=windTransformer.hv1 V  Winding2Connection=ee.enum.windingconnection.Yg  VRated2=4.16e3 V  CoreType=ee.enum.coretype.threelimb  pu_Rw1=windTransformer.windingResistance/20  pu_Rw2=windTransformer.windingResistance/20  leakage_reactance_option=ee.enum.transformer_leakage.include  pu_Xl1=windTransformer.windingLekageReactance/20  pu_Xl2=windTransformer.windingLekageReactance/20  magnetizing_resistance_option=ee.enum.transformer_magnetizingResistance.exclude  pu_Rm=500  magnetizing_reactance_option=ee.enum.transformer_magnetizingReactance.exclude  saturation_option=ee.enum.transformer_saturation.exclude  pu_Xm=500  current_data=[0, .002, 1, 2]  magnetic_flux_data=[0, 1.2, 1.5, 1.51]  pu_X0=windTransformer.zeroSequenceReactance  i1_specify=off  i1_priority=None  i1=[0, 0, 0] A  i1_nominal_specify=off  i1_nominal_value=1  i1_nominal_unit=A  i2_specify=off  i2_priority=None  i2=[0, 0, 0] A  i2_nominal_specify=off  i2_nominal_value=1  i2_nominal_unit=A  phi_specify=off  phi_priority=None  phi=[0, 0, 0]  phi_nominal_specify=off  phi_nominal_value=1  phi_nominal_unit=1  power_dissipated_specify=off  power_dissipated_priority=None  power_dissipated=0 W  power_dissipated_nominal_specify=off  power_dissipated_nominal_value=1  power_dissipated_nominal_unit=W
      settings: InternalSimscapePortConfiguration="{\"Bottom\":[],\"Left\":[{\"id\":\"N1\",\"label\":\"~1\",\"type\":\"foundation.electrical.three_phase\"}],\"Right\":[{\"id\":\"N2\",\"label\":\"~2\",\"type\":\"foundation.electrical.three_phase\"}],\"Top\":[]}"
  Controlled Current Source (Three-Phase) : ee_lib/Sources/Controlled Current Source (Three-Phase)  input_option=ee.enum.inputType.instantaneous  FRated=60 Hz
      settings: InternalSimscapePortConfiguration="{\"Bottom\":[],\"Left\":[{\"id\":\"S\",\"label\":\"S\",\"type\":\"input\"},{\"id\":\"n\",\"label\":\"n\",\"type\":\"foundation.electrical.electrical\"}],\"Right\":[{\"id\":\"N\",\"label\":\"~\",\"type\":\"foundation.electrical.three_phase\"}],\"Top\":[]}"
  Current Sensor (Three-Phase) : ee_lib/Sensors & Transducers/Current Sensor (Three-Phase)
  Electrical Reference : fl_lib/Electrical/Electrical Elements/Electrical Reference
  PLL & Measurements : Subsystem
      settings: PortSchema="{\"entries\":[{\"content\":{\"sides\":[{\"content\":{\"connectorIds\":[\"Out1\",\"In1\",\"In2\"]},\"type\":\"ConnectorPlacement.EquallySpacedRectSide\",\"uuid\":\"76485780-20fe-4fcf-8224-69648da6ed2a\"},{\"content\":{\"side\":\"RIGHT\"},\"type\":\"ConnectorPlacement.EquallySpacedRectSide\",\"uuid\":\"f19a6390-e634-42c7-8d46-4cd80cbab182\"},{\"content\":{\"side\":\"TOP\"},\"type\":\"ConnectorPlacement.EquallySpacedRectSide\",\"uuid\":\"87682f72-1844-428e-be70-ad7ca3191ee3\"}]},\"type\":\"ConnectorPlacement.EquallySpacedConnector\",\"uuid\":\"f2136b07-48ec-402b-adb3-18c0bac2157c\"}],\"packageUris\":[\"http://schema.mathworks.com/mf0/Connector/R2020b\"],\"version\":\"1.0\"}"
      mask Display: image('measurements.png'); % Use "Edit Image" on toolstrip to change.
  POI : ee_lib/Sensors & Transducers/Current and Voltage Sensor (Three-Phase)  vMeasurementType=ee.enum.vmeasurement.lg  outputUnit=ee.enum.unit.pu  SRated=base.mVA A*V  VRated=base.kV V  I_specify=off  I_priority=None  I=[0, 0, 0] A  I_nominal_specify=off  I_nominal_value=1  I_nominal_unit=A  V_specify=off  V_priority=None  V=[0, 0, 0] V  V_nominal_specify=off  V_nominal_value=1  V_nominal_unit=V
      settings: InternalSimscapePortConfiguration="{\"Bottom\":[],\"Left\":[{\"id\":\"N1\",\"label\":\"~1\",\"type\":\"foundation.electrical.three_phase\"}],\"Right\":[{\"id\":\"V_output\",\"label\":\"V\",\"type\":\"output\"},{\"id\":\"I_output\",\"label\":\"I\",\"type\":\"output\"},{\"id\":\"N2\",\"label\":\"~2\",\"type\":\"foundation.electrical.three_phase\"}],\"Top\":[]}"
  PS Gain : fl_lib/Physical Signals/Functions/PS Gain  gain=2
  PS-Simulink Converter{,1..2,4} (4 alike) : nesl_utility/PS-Simulink Converter  PhysicalDomain=network_engine_domain  SubClassName=ps_output  LeftPortType=input  RightPortType=output  PseudoPeriodic=off  Frequencies=[]  VectorFormat=inherit  Unit=inherit  AffineConversion=off
  Power Sensor (Three-Phase) : ee_lib/Sensors & Transducers/Power Sensor (Three-Phase)  load_type=ee.enum.passive.type_balanced.balanced  f0=60 Hz
      settings: InternalSimscapePortConfiguration="{\"Bottom\":[],\"Left\":[{\"id\":\"N1\",\"label\":\"~1\",\"type\":\"foundation.electrical.three_phase\"}],\"Right\":[{\"id\":\"N2\",\"label\":\"~2\",\"type\":\"foundation.electrical.three_phase\"}],\"Top\":[{\"id\":\"Pm\",\"label\":\"P\",\"type\":\"output\"},{\"id\":\"Qm\",\"label\":\"Q\",\"type\":\"output\"}]}"
  Wind Farm1 : Subsystem
  abc : PMIOPort  Side=Right
  P : Outport
  Q : Outport  Port=2
  wires:
  PS-Simulink Converter4/1 -> PLL & Measurements/2(Ig)  "Iabc"
  PS-Simulink Converter1/1 -> PLL & Measurements/1(V)  "Vabc"
  PS-Simulink Converter2/1 -> Q/1  "Q(RES)"
  PLL & Measurements/1(Vbus) -> Wind Farm1/1(Vbus)
  PS-Simulink Converter/1 -> P/1  "P(RES)"
  connections:
  PS-Simulink Converter4/LConn1 -- POI/RConn2
  Power Sensor (Three-Phase)/LConn3 -- PS-Simulink Converter2/LConn1
  Power Sensor (Three-Phase)/RConn1 -- POI/LConn1
  Power Sensor (Three-Phase)/LConn2 -- PS-Simulink Converter/LConn1
  PS-Simulink Converter1/LConn1 -- POI/RConn1
  32.6/4.16 kV/RConn1 -- POI/RConn3
  Wind Farm1/RConn1 -- Power Sensor (Three-Phase)/LConn1
  Current Sensor (Three-Phase)/LConn1 -- 32.6/4.16 kV/LConn1
  Current Sensor (Three-Phase)/RConn2 -- Controlled Current Source (Three-Phase)/RConn1 -- abc/RConn1
  PS Gain/LConn1 -- Current Sensor (Three-Phase)/RConn1
  Electrical Reference/LConn1 -- Controlled Current Source (Three-Phase)/LConn2
  PS Gain/RConn1 -- Controlled Current Source (Three-Phase)/LConn1

== system VSCHVDCunit/Cables/Idcnr ==
  Current Sensor : fl_lib/Electrical/Electrical Sensors/Current Sensor
  PS-Simulink Converter : nesl_utility/PS-Simulink Converter  PhysicalDomain=network_engine_domain  SubClassName=ps_output  LeftPortType=input  RightPortType=output  PseudoPeriodic=off  Frequencies=[]  VectorFormat=1-D array  Unit=A  AffineConversion=off
  + : PMIOPort  Side=Left
  - : PMIOPort  Port=2  Side=Right
  i : Outport
  wires:
  PS-Simulink Converter/1 -> i/1
  connections:
  -/RConn1 -- Current Sensor/RConn2
  Current Sensor/LConn1 -- +/RConn1
  PS-Simulink Converter/LConn1 -- Current Sensor/RConn1

== system VSCHVDCunit/Cables/Idcns ==
  Current Sensor : fl_lib/Electrical/Electrical Sensors/Current Sensor
  PS-Simulink Converter : nesl_utility/PS-Simulink Converter  PhysicalDomain=network_engine_domain  SubClassName=ps_output  LeftPortType=input  RightPortType=output  PseudoPeriodic=off  Frequencies=[]  VectorFormat=1-D array  Unit=A  AffineConversion=off
  + : PMIOPort  Side=Left
  - : PMIOPort  Port=2  Side=Right
  i : Outport
  wires:
  PS-Simulink Converter/1 -> i/1
  connections:
  PS-Simulink Converter/LConn1 -- Current Sensor/RConn1
  Current Sensor/LConn1 -- +/RConn1
  -/RConn1 -- Current Sensor/RConn2

== system VSCHVDCunit/Cables/Idcpr ==
  Current Sensor : fl_lib/Electrical/Electrical Sensors/Current Sensor
  PS-Simulink Converter : nesl_utility/PS-Simulink Converter  PhysicalDomain=network_engine_domain  SubClassName=ps_output  LeftPortType=input  RightPortType=output  PseudoPeriodic=off  Frequencies=[]  VectorFormat=1-D array  Unit=A  AffineConversion=off
  + : PMIOPort  Side=Left
  - : PMIOPort  Port=2  Side=Right
  i : Outport
  wires:
  PS-Simulink Converter/1 -> i/1
  connections:
  PS-Simulink Converter/LConn1 -- Current Sensor/RConn1
  Current Sensor/LConn1 -- +/RConn1
  -/RConn1 -- Current Sensor/RConn2

== system VSCHVDCunit/Cables/Idcps ==
  Current Sensor : fl_lib/Electrical/Electrical Sensors/Current Sensor
  PS-Simulink Converter : nesl_utility/PS-Simulink Converter  PhysicalDomain=network_engine_domain  SubClassName=ps_output  LeftPortType=input  RightPortType=output  PseudoPeriodic=off  Frequencies=[]  VectorFormat=1-D array  Unit=A  AffineConversion=off
  + : PMIOPort  Side=Left
  - : PMIOPort  Port=2  Side=Right
  i : Outport
  wires:
  PS-Simulink Converter/1 -> i/1
  connections:
  -/RConn1 -- Current Sensor/RConn2
  Current Sensor/LConn1 -- +/RConn1
  PS-Simulink Converter/LConn1 -- Current Sensor/RConn1

== system VSCHVDCunit/Cables/Vdcnr ==
  PS-Simulink Converter : nesl_utility/PS-Simulink Converter  PhysicalDomain=network_engine_domain  SubClassName=ps_output  LeftPortType=input  RightPortType=output  PseudoPeriodic=off  Frequencies=[]  VectorFormat=1-D array  Unit=V  AffineConversion=off
  Voltage Sensor : fl_lib/Electrical/Electrical Sensors/Voltage Sensor
  + : PMIOPort  Side=Left
  - : PMIOPort  Port=2  Side=Right
  v : Outport
  wires:
  PS-Simulink Converter/1 -> v/1
  connections:
  PS-Simulink Converter/LConn1 -- Voltage Sensor/RConn1
  Voltage Sensor/RConn2 -- -/RConn1
  Voltage Sensor/LConn1 -- +/RConn1

== system VSCHVDCunit/Cables/Vdcns ==
  PS-Simulink Converter : nesl_utility/PS-Simulink Converter  PhysicalDomain=network_engine_domain  SubClassName=ps_output  LeftPortType=input  RightPortType=output  PseudoPeriodic=off  Frequencies=[]  VectorFormat=1-D array  Unit=V  AffineConversion=off
  Voltage Sensor : fl_lib/Electrical/Electrical Sensors/Voltage Sensor
  + : PMIOPort  Side=Left
  - : PMIOPort  Port=2  Side=Right
  v : Outport
  wires:
  PS-Simulink Converter/1 -> v/1
  connections:
  Voltage Sensor/LConn1 -- +/RConn1
  Voltage Sensor/RConn2 -- -/RConn1
  PS-Simulink Converter/LConn1 -- Voltage Sensor/RConn1

== system VSCHVDCunit/Cables/Vdcpr ==
  PS-Simulink Converter : nesl_utility/PS-Simulink Converter  PhysicalDomain=network_engine_domain  SubClassName=ps_output  LeftPortType=input  RightPortType=output  PseudoPeriodic=off  Frequencies=[]  VectorFormat=1-D array  Unit=V  AffineConversion=off
  Voltage Sensor : fl_lib/Electrical/Electrical Sensors/Voltage Sensor
  + : PMIOPort  Side=Left
  - : PMIOPort  Port=2  Side=Right
  v : Outport
  wires:
  PS-Simulink Converter/1 -> v/1
  connections:
  Voltage Sensor/LConn1 -- +/RConn1
  Voltage Sensor/RConn2 -- -/RConn1
  PS-Simulink Converter/LConn1 -- Voltage Sensor/RConn1

== system VSCHVDCunit/Cables/Vdcps ==
  PS-Simulink Converter : nesl_utility/PS-Simulink Converter  PhysicalDomain=network_engine_domain  SubClassName=ps_output  LeftPortType=input  RightPortType=output  PseudoPeriodic=off  Frequencies=[]  VectorFormat=1-D array  Unit=V  AffineConversion=off
  Voltage Sensor : fl_lib/Electrical/Electrical Sensors/Voltage Sensor
  + : PMIOPort  Side=Left
  - : PMIOPort  Port=2  Side=Right
  v : Outport
  wires:
  PS-Simulink Converter/1 -> v/1
  connections:
  PS-Simulink Converter/LConn1 -- Voltage Sensor/RConn1
  Voltage Sensor/RConn2 -- -/RConn1
  Voltage Sensor/LConn1 -- +/RConn1

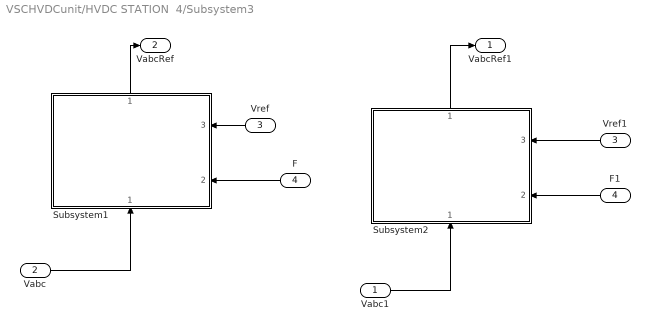
== system VSCHVDCunit/HVDC STATION  4/Subsystem3 ==
  Vabc1 : Inport
  Vabc : Inport  Port=2
  Vref : Inport  Port=3
  F : Inport  Port=4
  F1 : InportShadow  Port=4
  Subsystem1 : Subsystem  ReferencedSubsystem=WFController  Kpv=offshoregfm.kvp  Kiv=offshoregfm.kvi  Kpicd=offshoregfm.kip  Kiicd=offshoregfm.kii  Kpicq=offshoregfm.kip  Kiicq=offshoregfm.kii  mVAbase=base.mVA  frequency=Grid.frequency  zBase=base.z  iMax=offshoregfm.Imax  L=HVDC.L/5  Kv=base.kV1
      settings: PortSchema="{\"entries\":[{\"content\":{\"sides\":[{\"content\":{\"connectorIds\":[\"In1\"]},\"type\":\"ConnectorPlacement.EquallySpacedRectSide\",\"uuid\":\"46af9a47-930e-4d26-bbce-c3520b6c2749\"},{\"content\":{\"connectorIds\":[\"Out1\"],\"side\":\"RIGHT\"},\"type\":\"ConnectorPlacement.EquallySpacedRectSide\",\"uuid\":\"6339fe7c-3981-41e7-9f19-cda16be41a14\"},{\"content\":{\"side\":\"TOP\"},\"type\":\"ConnectorPlacement.EquallySpacedRectSide\",\"uuid\":\"d1729033-563f-49aa-8053-bb4cbe37e0ab\"},{\"content\":{\"connectorIds\":[\"In2\",\"In3\"],\"side\":\"BOTTOM\"},\"type\":\"ConnectorPlacement.EquallySpacedRectSide\",\"uuid\":\"30ea6182-355c-4132-b992-4839827195ad\"}]},\"type\":\"ConnectorPlacement.EquallySpacedConnector\",\"uuid\":\"fc0bd660-6248-4e50-8baf-5497ce638304\"}],\"packageUris\":[\"http://schema.mathworks.com/mf0/Connector/R2020b\"],\"version\":\"1.0\"}"
  Subsystem2 : Subsystem  ReferencedSubsystem=WFController  Kpv=offshoregfm.kvp  Kiv=offshoregfm.kvi  Kpicd=offshoregfm.kip  Kiicd=offshoregfm.kii  Kpicq=offshoregfm.kip  Kiicq=offshoregfm.kii  mVAbase=base.mVA  frequency=Grid.frequency  zBase=base.z  iMax=offshoregfm.Imax  L=HVDC.L/5  Kv=base.kV1
      settings: PortSchema="{\"entries\":[{\"content\":{\"sides\":[{\"content\":{\"connectorIds\":[\"In1\"]},\"type\":\"ConnectorPlacement.EquallySpacedRectSide\",\"uuid\":\"46af9a47-930e-4d26-bbce-c3520b6c2749\"},{\"content\":{\"connectorIds\":[\"Out1\"],\"side\":\"RIGHT\"},\"type\":\"ConnectorPlacement.EquallySpacedRectSide\",\"uuid\":\"6339fe7c-3981-41e7-9f19-cda16be41a14\"},{\"content\":{\"side\":\"TOP\"},\"type\":\"ConnectorPlacement.EquallySpacedRectSide\",\"uuid\":\"d1729033-563f-49aa-8053-bb4cbe37e0ab\"},{\"content\":{\"connectorIds\":[\"In2\",\"In3\"],\"side\":\"BOTTOM\"},\"type\":\"ConnectorPlacement.EquallySpacedRectSide\",\"uuid\":\"30ea6182-355c-4132-b992-4839827195ad\"}]},\"type\":\"ConnectorPlacement.EquallySpacedConnector\",\"uuid\":\"fc0bd660-6248-4e50-8baf-5497ce638304\"}],\"packageUris\":[\"http://schema.mathworks.com/mf0/Connector/R2020b\"],\"version\":\"1.0\"}"
  Vref1 : InportShadow  Port=3
  VabcRef1 : Outport
  VabcRef : Outport  Port=2
  wires:
  Vabc/1 -> Subsystem1/1
  Vref/1 -> Subsystem1/3
  F/1 -> Subsystem1/2
  Vabc1/1 -> Subsystem2/1
  F1/1 -> Subsystem2/2
  Vref1/1 -> Subsystem2/3
  Subsystem1/1 -> VabcRef/1
  Subsystem2/1 -> VabcRef1/1

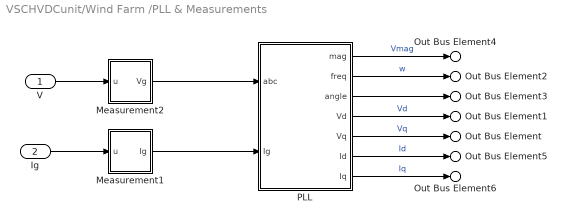
== system VSCHVDCunit/Wind Farm /PLL & Measurements ==
  V : Inport
  Ig : Inport  Port=2
  Measurement1 : Subsystem
  Measurement2 : Subsystem
  PLL : Subsystem
  Out Bus Element : Outport  PortName=Vbus  Element=Vq
  Out Bus Element1 : Outport  PortName=Vbus  Element=Vd
  Out Bus Element2 : Outport  PortName=Vbus  Element=w
  Out Bus Element3 : Outport  PortName=Vbus  Element=Theta
  Out Bus Element4 : Outport  PortName=Vbus  Element=Vmag
  Out Bus Element5 : Outport  PortName=Vbus  Element=Id
  Out Bus Element6 : Outport  PortName=Vbus  Element=Iq
  wires:
  V/1 -> Measurement2/1(u)
  PLL/2(freq) -> Out Bus Element2/1  "w"
  PLL/5(Vq) -> Out Bus Element/1  "Vq"
  PLL/3(angle) -> Out Bus Element3/1
  PLL/4(Vd) -> Out Bus Element1/1  "Vd"
  Measurement2/1(Vg) -> PLL/1(abc)
  PLL/1(mag) -> Out Bus Element4/1  "Vmag"
  Measurement1/1(Ig) -> PLL/2(Ig)
  Ig/1 -> Measurement1/1(u)
  PLL/7(Iq) -> Out Bus Element6/1  "Iq"
  PLL/6(Id) -> Out Bus Element5/1  "Id"
